simulink model "simulink_tesis"  (R2018b)
settings: Solver=VariableStepAuto  StartTime=0.0  StopTime=20  RelTol=1e-3
values from neighbouring files (symbols this model uses):
  X0 = [-0.75 0.25]    [run_only_this_file.m]
libraries: truetime x4, simulink x1
settings Model: Creator=Asus ROG  LastModifiedBy=Asus ROG
settings DataIOCC: Refine=5
settings SFSimCC: SimUseLocalCustomCode=off
settings RTWCC: RTWUseLocalCustomCode=off
settings CodeAppCC: StateflowObjectComments=on
settings ConfigComp: DVTestSuiteOptimization=CombinedObjectives (Nonlinear Extended)  DVDetectOutOfBounds=on

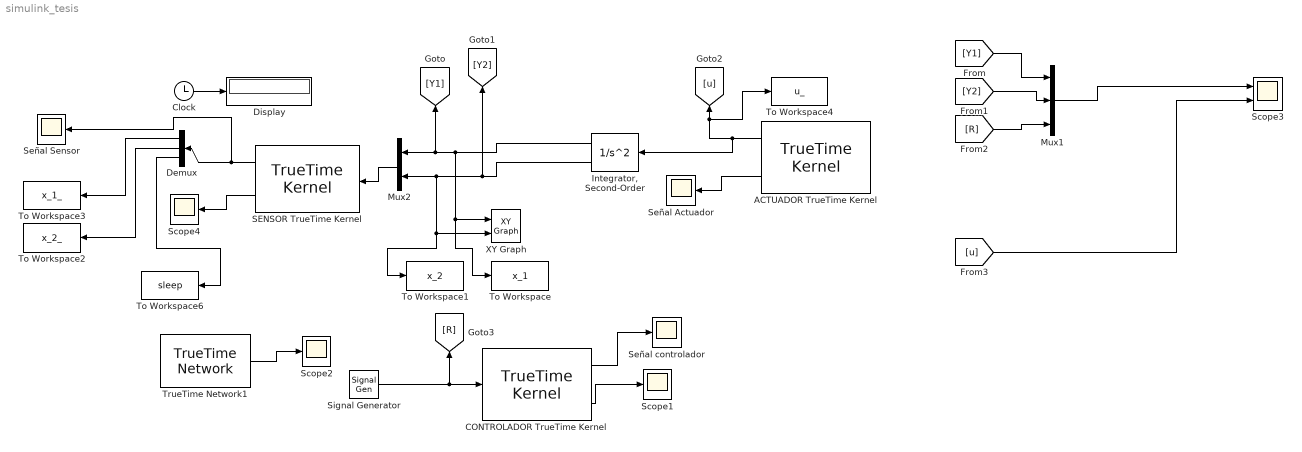
== system simulink_tesis ==
  ACTUADOR TrueTime Kernel : truetime/TrueTime Kernel  sfun=actuador_node  args=[]  ninputsoutputs=[0 1]  ntriggers=0  trigtype=falling  nwnodenbr=[2]  clockoffsetdrift=[0 0]  schedoutput=on  battery=off  poweroutput=off  label=1: 2
  CONTROLADOR TrueTime Kernel : truetime/TrueTime Kernel  sfun=control_node  args=[]  ninputsoutputs=[1 1]  ntriggers=0  trigtype=falling  nwnodenbr=3  clockoffsetdrift=[0 0]  schedoutput=on  battery=off  poweroutput=off  label=1: 3
  Clock : Clock
  Demux : Demux  Outputs=3
  Display : Display
  "Integrator, Second-Order" : SecondOrderIntegrator  ICX=X0(1,1)  ICDXDT=X0(1,2)
  Mux1 : Mux  Inputs=3
  Mux2 : Mux  Inputs=2
  SENSOR TrueTime Kernel : truetime/TrueTime Kernel  sfun=sensor_node  args=[]  ninputsoutputs=[2 3]  ntriggers=0  trigtype=falling  nwnodenbr=1  clockoffsetdrift=[0 0]  schedoutput=on  battery=off  poweroutput=off  label=1: 1
  Scope1 : Scope
  Scope2 : Scope
  Scope3 : Scope  NumInputPorts=2
  Scope4 : Scope
  Señal Actuador : Scope
  Señal Sensor : Scope
  Señal controlador : Scope
  Signal Generator : SignalGenerator  Amplitude=0.2  Frequency=10  Units=rad/sec
  To Workspace : ToWorkspace  VariableName=x_1  SampleTime=-1
      settings: Decimation=2  Save2DSignal=2-D array (concatenate along first dimension)
  To Workspace1 : ToWorkspace  VariableName=x_2  SampleTime=-1
      settings: Decimation=2  Save2DSignal=2-D array (concatenate along first dimension)
  To Workspace2 : ToWorkspace  VariableName=x_2_  SampleTime=-1
      settings: Decimation=2
  To Workspace3 : ToWorkspace  VariableName=x_1_  SampleTime=-1
      settings: Decimation=2
  To Workspace4 : ToWorkspace  VariableName=u_  SampleTime=-1
      settings: Decimation=2
  To Workspace6 : ToWorkspace  VariableName=sleep  SaveFormat=Timeseries  SampleTime=-1
      settings: Decimation=2
  TrueTime Network1 : truetime/TrueTime Network  nwtype=CSMA/AMP (CAN)  nwnbr=1  nnodes=3  rate=10000000  minsize=80  lossprob=0  seed=0  bandwidths=[0.5 0.5]  slotsize=512  schedule=[1 1 2]  memsize=80000  buftype=Common buffer  overflow=Retransmit  dynSchedule=0  miniSlotSize=0  NIT=0  QSortMode=FIFO  sync=0  irtSchedule=0  nrtLength=0  nodeGraph=0  scheduleoutput=on
  XY Graph : simulink/Sinks/XY Graph  xmin=-1  xmax=1  ymin=-1  ymax=1  st=-1
  wires:
  ACTUADOR TrueTime Kernel/2 -> Señal Actuador/1
  CONTROLADOR TrueTime Kernel/2 -> Scope1/1
  TrueTime Network1/1 -> Scope2/1
  Signal Generator/1 -> [R], CONTROLADOR TrueTime Kernel/1
  SENSOR TrueTime Kernel/2 -> Scope4/1
  Clock/1 -> Display/1
  Mux1/1 -> Scope3/1
  [Y2] -> Mux1/2
  [Y1] -> Mux1/1
  [R] -> Mux1/3
  ACTUADOR TrueTime Kernel/1 -> "Integrator, Second-Order"/1, To Workspace4/1, [u]
  CONTROLADOR TrueTime Kernel/1 -> Señal controlador/1
  Mux2/1 -> SENSOR TrueTime Kernel/1
  [u] -> Scope3/2
  "Integrator, Second-Order"/1 -> To Workspace/1, XY Graph/1, [Y1], Mux2/1
  "Integrator, Second-Order"/2 -> [Y2], To Workspace1/1, XY Graph/2, Mux2/2
  SENSOR TrueTime Kernel/1 -> Señal Sensor/1, Demux/1
  Demux/1 -> To Workspace3/1
  Demux/2 -> To Workspace2/1
  Demux/3 -> To Workspace6/1
